simulink model "mod8"  (R2018b)
settings: Solver=FixedStepAuto  StartTime=0.0  StopTime=300  FixedStep=1e-2  RelTol=1e-3  EnableMultiTasking=on
values from neighbouring files (symbols this model uses):
  d = 0.5    [mod1s.m]
  h = 4    [mod1s.m]
  K = 19    [mod1s.m]
  k1 = 3    [mod1s.m]
  k2 = 40    [mod1s.m]
  T = 29    [mod1s.m]
settings Model: Creator=user  LastModifiedBy=ogure
settings SolverCC: SolverResetMethod=Robust
settings DataIOCC: LimitDataPoints=on  SaveFormat=Array  SaveOutput=off  OutputSaveName=X,X1,X2,X3,X4,L,H
settings OptimizationCC: LifeSpan=inf
settings DebuggingCC: SolverPrmCheckMsg=warning  SFUnexpectedBacktrackingDiag=warning  SFNoUnconditionalDefaultTransitionDiag=warning  SFExecutionAtInitializationDiag=none
settings HardwareCC: ProdBitPerPointer=32  ProdBitPerSizeT=32  ProdBitPerPtrDiffT=32  ProdLargestAtomicFloat=None  ProdIntDivRoundTo=Undefined  ProdEndianess=Unspecified  ProdWordSize=32  ProdHWDeviceType=32-bit Generic
settings ModelReferenceCC: PropagateSignalLabelsOutOfModel=off
settings SFSimCC: SimUseLocalCustomCode=off
settings RTWCC: RTWUseLocalCustomCode=off
settings CodeAppCC: StateflowObjectComments=on
settings GRTTargetCC: TargetLangStandard=C89/C90 (ANSI)  GeneratePreprocessorConditionals=Disable all
settings ConfigComp: CovMetricSettings=dw  CovHtmlReporting=on  CovSaveCumulativeToWorkspaceVar=on  CovSaveSingleToWorkspaceVar=on  CovExternalEMLEnable=off  CovSFcnEnable=off

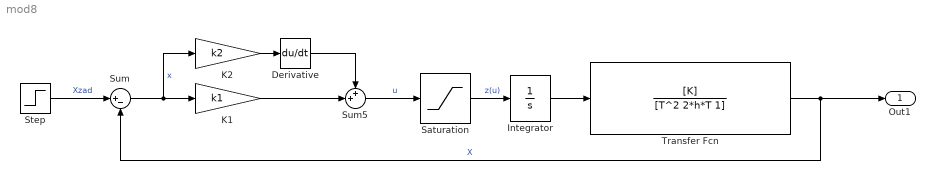
== system mod8 ==
  Derivative : Derivative  CoefficientInTFapproximation=0.00000001
  Integrator : Integrator
  K1 : Gain  Gain=k1
  "K2 " : Gain  Gain=k2
  Saturation : Saturate  UpperLimit=d  LowerLimit=-d
  Step : Step  SampleTime=0
  Sum : Sum  Inputs=|+-
  Sum5 : Sum  Inputs=++|
  Transfer Fcn : TransferFcn  Numerator=[K]  Denominator=[T^2 2*h*T 1]
  Out1 : Outport  SignalName=X
  wires:
  Transfer Fcn/1 -> Sum/2, Out1/1  "X"
  Integrator/1 -> Transfer Fcn/1
  Step/1 -> Sum/1  "Xzad"
  Sum5/1 -> Saturation/1  "u"
  Saturation/1 -> Integrator/1  "z(u)"
  Derivative/1 -> Sum5/1
  K1/1 -> Sum5/2
  Sum/1 -> K1/1, "K2 "/1  "x"
  "K2 "/1 -> Derivative/1
